simulink model "flightControlSystem"  (R2020b)
settings: Solver=ode3  StartTime=0  StopTime=inf  FixedStep=Ts  RelTol=1e-3  EnableMultiTasking=on
model workspace (MAT data in the model file):
  bwmaskcircle = Simulink.Parameter
  bwmaskcircle.Value = [0 0 0 0 0 0 0 0 0 0 0 0 ... (19200 elements, 120x160)]
  bwmaskcircle.DataType = 'boolean'
  bwmaskcircle.Dimensions = [120 160]
  bwmaskcorner = Simulink.Parameter
  bwmaskcorner.Value = [1 1 1 1 1 1 1 1 1 1 1 1 ... (19200 elements, 120x160)]
  bwmaskcorner.DataType = 'auto'
  bwmaskcorner.Dimensions = [120 160]
  bwmaskland = Simulink.Parameter
  bwmaskland.Value = [0 0 0 0 0 0 0 0 0 0 0 0 ... (19200 elements, 120x160)]
  bwmaskland.DataType = 'auto'
  bwmaskland.Dimensions = [120 160]
  bwmaskleft = Simulink.Parameter
  bwmaskleft.Value = [0 0 0 0 0 0 0 0 0 0 0 0 ... (19200 elements, 120x160)]
  bwmaskleft.DataType = 'auto'
  bwmaskleft.Dimensions = [120 160]
  bwmaskleftmatrix = [0 0 0 0 0 0 0 0 0 0 0 0 ... (6912000 elements, 120x160x360)]
  bwmaskpathtrianglematrix = [0 0 0 0 0 0 0 0 0 0 0 0 ... (6931200 elements, 120x160x361)]
  bwmaskpathtrianglematrix360 = [0 0 0 0 0 0 0 0 0 0 0 0 ... (6912000 elements, 120x160x360)]
  bwmaskright = Simulink.Parameter
  bwmaskright.Value = [0 0 0 0 0 0 0 0 0 0 0 0 ... (19200 elements, 120x160)]
  bwmaskright.DataType = 'auto'
  bwmaskright.Dimensions = [120 160]
  bwmaskrightmatrix = [0 0 0 0 0 0 0 0 0 0 0 0 ... (6912000 elements, 120x160x360)]
  bwmasksquare = Simulink.Parameter
  bwmasksquare.Value = [0 0 0 0 0 0 0 0 0 0 0 0 ... (19200 elements, 120x160)]
  bwmasksquare.DataType = 'auto'
  bwmasksquare.Dimensions = [120 160]
  bwmasktrapezoid = Simulink.Parameter
  bwmasktrapezoid.Value = [0 0 0 0 0 0 0 0 0 0 0 0 ... (19200 elements, 120x160)]
  bwmasktrapezoid.DataType = 'auto'
  bwmasktrapezoid.Dimensions = [120 160]
  bwmasktrapezoidmatrix = [0 0 0 0 0 0 0 0 0 0 0 0 ... (6931200 elements, 120x160x361)]
  bwmasktrapezoidmatrix360 = [0 0 0 0 0 0 0 0 0 0 0 0 ... (6912000 elements, 120x160x360)]
  bwmasktrapezoidmatrixold = [0 0 0 0 0 0 0 0 0 0 0 0 ... (6912000 elements, 120x160x360)]
  bwmasktraveled = Simulink.Parameter
  bwmasktraveled.Value = [1 1 1 1 1 1 1 1 1 1 1 1 ... (19200 elements, 120x160)]
  bwmasktraveled.DataType = 'auto'
  bwmasktraveled.Dimensions = [120 160]
  bwmasktraveledmatrix = [1 1 1 1 1 1 1 1 1 1 1 1 ... (6931200 elements, 120x160x361)]
  bwmasktraveledmatrix360 = [0 0 0 0 0 0 0 0 0 0 0 0 ... (6912000 elements, 120x160x360)]
  bwmasktraveledpast = Simulink.Parameter
  bwmasktraveledpast.Value = [1 1 1 1 1 1 1 1 1 1 1 1 ... (19200 elements, 120x160)]
  bwmasktraveledpast.DataType = 'auto'
  bwmasktraveledpast.Dimensions = [120 160]
undefined symbols (not defined in the file): bwmaskpathtrianglematrixmatlab, bwmasktrapezoidmatrixmatlab, bwmasktraveledmatrixmatlab, codertarget, Controller, DiscIntNeverNeededParam, Discrete, Estimator, g, gray, init, orient_ref, pos_ref, Sensors, strel, Time, Ts, var_acc_angle_N, var_bias_gyr_N, var_gyro_p_N, Vehicle
libraries: simulink x40, pid_lib x5, ctrlSharedLib x4, sharedtransform x3, visiontextngfix x3, visionstatistics x2, visionmorphops x2, parrotlib x1, simulink_extras x1
(part 1 of 4)
settings Model: ExtModeTrigDuration=80  OrderedModelArguments=off  Creator=The MathWorks, Inc.  LastModifiedBy=eber_
settings DataIOCC: LimitDataPoints=on  SaveFormat=StructureWithTime  SaveOutput=off  DSMLogging=off  SaveTime=off  ReturnWorkspaceOutputs=off
settings OptimizationCC: BlockReduction=off  EnhancedBackFolding=on  PassReuseOutputArgsThreshold=0  MaxStackSize=64  OptimizeBlockOrder=speed  DifferentSizesBufferReuse=on
settings DebuggingCC: AlgebraicLoopMsg=none  ParameterPrecisionLossMsg=none  ParameterTunabilityLossMsg=error  UnconnectedInputMsg=none  UnconnectedOutputMsg=none  UnconnectedLineMsg=none  BusObjectLabelMismatch=error  PregeneratedLibrarySubsystemCodeDiagnostic=none  SFUnexpectedBacktrackingDiag=warning  SFNoUnconditionalDefaultTransitionDiag=warning  SFExecutionAtInitializationDiag=none  ArithmeticOperatorsInVariantConditions=warning
settings HardwareCC: ProdBitPerPointer=32  ProdBitPerSizeT=32  ProdBitPerPtrDiffT=32  ProdLargestAtomicInteger=Long  ProdWordSize=32  ProdHWDeviceType=ARM Compatible->ARM 9  UseEmbeddedCoderFeatures=off
settings ModelReferenceCC: ModelReferenceNumInstancesAllowed=Single  PropagateSignalLabelsOutOfModel=off
settings SFSimCC: SimUseLocalCustomCode=off  MATLABDynamicMemAlloc=off  CustomCodeUndefinedFunction=UseInterfaceOnly
settings RTWCC: Description=Embedded Coder  SystemTargetFile=ert.tlc  HardwareBoard=PARROT Mambo  TemplateMakefile=ert_default_tmf  RTWUseLocalCustomCode=off  Toolchain=Sourcery G++ Lite GNU Toolchain for Drones
settings CodeAppCC: ForceParamTrailComments=on  MaxIdLength=63  OperatorAnnotations=on  MangleLength=10
settings ERTTargetCC: CombineOutputUpdateFcns=off  ERTCustomFileBanners=off  SupportContinuousTime=on  SupportNonInlinedSFcns=on  RemoveResetFunc=off  ModelStepFunctionPrototypeControlCompliant=off
settings ConfigComp: CovMetricSettings=dw  CovSaveCumulativeToWorkspaceVar=on  CovSaveSingleToWorkspaceVar=on  CovExternalEMLEnable=off  CovSFcnEnable=off

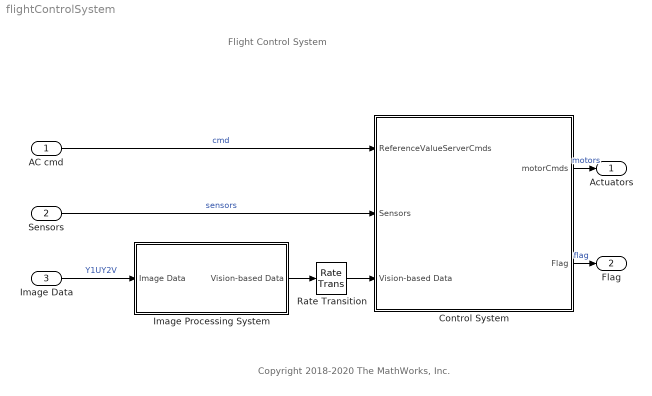
== system flightControlSystem ==
  note: Copyright 2018-2020 The MathWorks, Inc.
  note: Flight Control System
  AC cmd : Inport  OutDataTypeStr=Bus: CommandBus  BusOutputAsStruct=on
  Sensors : Inport  Port=2  OutDataTypeStr=Bus: SensorsBus  BusOutputAsStruct=on
  Image Data : Inport  Tag=IP_IN  InitFcn=codertarget.parrot.internal.inportCallback(gcb);  Port=3  OutDataTypeStr=uint8  PortDimensions=[4 9600]  BusOutputAsStruct=on
  Control System : Subsystem  InitFcn=codertarget.parrot.internal.fcsSubsystemCallback(gcb);  TreatAsAtomicUnit=on  SystemSampleTime=Ts
  Image Processing System : Subsystem  Tag=IP_SUB  InitFcn=codertarget.parrot.internal.ipSubsystemCallback(gcb);  TreatAsAtomicUnit=on  SystemSampleTime=40*Ts  RTWFcnName=ImageFunction
      settings: RTWSystemCode=Inline  RTWFcnNameOpts=User specified
  Rate Transition : RateTransition  Deterministic=off
  Actuators : Outport  OutDataTypeStr=single  PortDimensions=4  VectorParamsAs1DForOutWhenUnconnected=off
  Flag : Outport  Port=2  OutDataTypeStr=uint8  PortDimensions=1  VectorParamsAs1DForOutWhenUnconnected=off
  wires:
  AC cmd/1 -> Control System/1(ReferenceValueServerCmds)  "cmd"
  Control System/1(motorCmds) -> Actuators/1  "motors"
  Sensors/1 -> Control System/2(Sensors)  "sensors"
  Control System/2(Flag) -> Flag/1  "flag"
  Image Data/1 -> Image Processing System/1(Image Data)  "Y1UY2V"
  Image Processing System/1(Vision-based Data) -> Rate Transition/1
  Rate Transition/1 -> Control System/3(Vision-based Data)
